simulink model "performace_controllore_Hinf"  (R2023b)
settings: Solver=VariableStepAuto  StartTime=0.0  StopTime=10.0  RelTol=1e-3
libraries: cstblocks x2
settings Model: Creator=roberto_ambrosino  LastModifiedBy=roberto_ambrosino

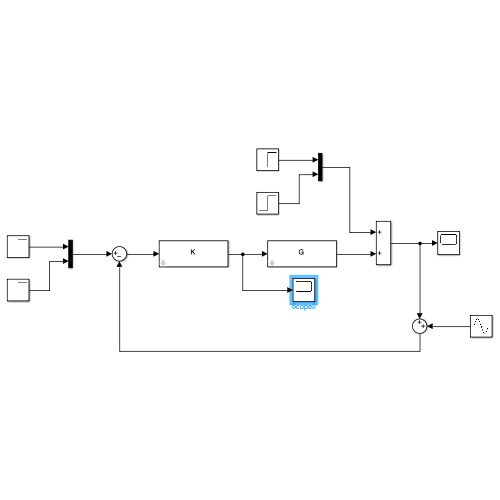
[thumbnail: Simulink's stored preview of the top-level diagram]
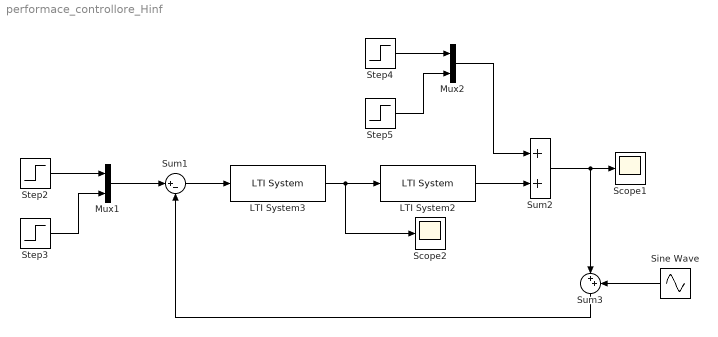
== system performace_controllore_Hinf ==
  LTI System2 : cstblocks/LTI System  sys=G  IC=[]  PadeOrder=0
  LTI System3 : cstblocks/LTI System  sys=K  IC=[]  PadeOrder=0
  Mux1 : Mux  Inputs=2
  Mux2 : Mux  Inputs=2
  Scope1 : Scope
  Scope2 : Scope
  Sine Wave : Sin  Amplitude=0  Frequency=100  SampleTime=0
  Step2 : Step  Time=0  After=2  SampleTime=0
  Step3 : Step  Time=0  SampleTime=0
  Step4 : Step  Time=0  After=0  SampleTime=0
  Step5 : Step  Time=0  After=0  SampleTime=0
  Sum1 : Sum  Inputs=|+-
  Sum2 : Sum
  Sum3 : Sum  Inputs=|++
  wires:
  Sum1/1 -> LTI System3/1
  Step3/1 -> Mux1/2
  LTI System3/1 -> Scope2/1, LTI System2/1
  Step2/1 -> Mux1/1
  Mux1/1 -> Sum1/1
  LTI System2/1 -> Sum2/2
  Sum2/1 -> Sum3/1, Scope1/1
  Step4/1 -> Mux2/1
  Step5/1 -> Mux2/2
  Mux2/1 -> Sum2/1
  Sine Wave/1 -> Sum3/2
  Sum3/1 -> Sum1/2
